simulink model "new5"  (R2025a)
settings: Solver=VariableStepAuto  StartTime=0.0  StopTime=20  RelTol=1e-3
undefined symbols (not defined in the file): g, Rs, Rsl, Rw, Ry
libraries: fl_lib x41, ee_lib x10, nesl_utility x10, slpidlib x3, spsFirstOrderFilterLib x2, spsabctodq0Lib x1
settings Model: SimulationMode=accelerator  Creator=maska  LastModifiedBy=maska

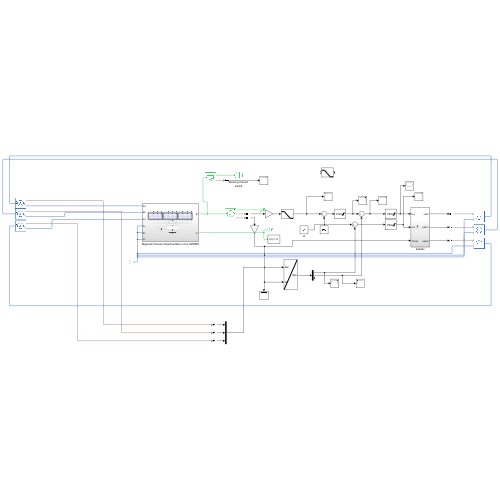
[thumbnail: Simulink's stored preview of the top-level diagram]
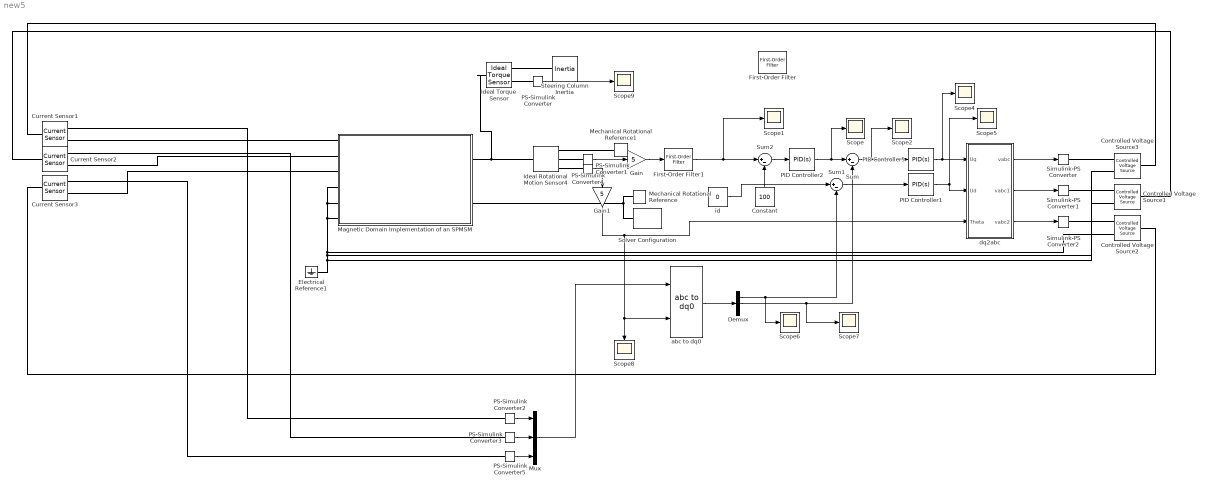
== system new5 ==
  Constant : Constant  Value=100
  Controlled Voltage Source1 : fl_lib/Electrical/Electrical Sources/Controlled Voltage Source
  Controlled Voltage Source2 : fl_lib/Electrical/Electrical Sources/Controlled Voltage Source
  Controlled Voltage Source3 : fl_lib/Electrical/Electrical Sources/Controlled Voltage Source
  Current Sensor1 : fl_lib/Electrical/Electrical Sensors/Current Sensor
  Current Sensor2 : fl_lib/Electrical/Electrical Sensors/Current Sensor
  Current Sensor3 : fl_lib/Electrical/Electrical Sensors/Current Sensor
  Demux : Demux  Outputs=3
  Electrical Reference1 : fl_lib/Electrical/Electrical Elements/Electrical Reference
  First-Order Filter : spsFirstOrderFilterLib/First-Order Filter  FilterType=Lowpass  Tc=0.05  Ts=0  Initialize=on  Vac_Init=[0, 0, 60]  Vdc_Init=0  PlotResponse=off  FreqRange="[0,  200,  1]"
  First-Order Filter1 : spsFirstOrderFilterLib/First-Order Filter  FilterType=Lowpass  Tc=0.1  Ts=0  Initialize=on  Vac_Init=[0, 0, 60]  Vdc_Init=0  PlotResponse=off  FreqRange="[0,  200,  1]"
  Gain : Gain  Gain=5
  Gain1 : Gain  Gain=5
  Ideal Rotational Motion Sensor4 : fl_lib/Mechanical/Mechanical Sensors/Ideal Rotational Motion Sensor  reference=foundation.enum.MeasurementReference.difference  acceleration_port=false  velocity_port=true  position_port=true  wrap_angle=false  offset=0 rad
  Ideal Torque Sensor : fl_lib/Mechanical/Mechanical Sensors/Ideal Torque Sensor
  Magnetic Domain Implementation of an SPMSM : Subsystem
  Mechanical Rotational Reference : fl_lib/Mechanical/Rotational Elements/Mechanical Rotational Reference
  Mechanical Rotational Reference1 : fl_lib/Mechanical/Rotational Elements/Mechanical Rotational Reference
  Mux : Mux  Inputs=3
  PID Controller1 : slpidlib/PID Controller  Controller=PID  Form=Parallel  TimeDomain=Continuous-time  UseExternalTs=off  SampleTime=-1  IntegratorMethod=Forward Euler  FilterMethod=Forward Euler  ControllerParametersSource=internal  P=1.3  I=0.3  UseKiTs=off  D=0  UseExternalDerivativeSource=off  N=100  UseFilter=on  TunerSelectOption=Transfer Function Based (PID Tuner App)  InitialConditionSource=internal  InitialConditionForIntegrator=0  InitialConditionForFilter=0  DifferentiatorICPrevScaledInput=0  ExternalReset=none  TrackingMode=off  Kt=1  LimitOutput=on  SatLimitsSource=internal  UpperSaturationLimit=1000  LowerSaturationLimit=-1000  LinearizeAsGain=on  AntiWindupMode=none  Kb=1  LimitIntegrator=off  UpperIntegratorSaturationLimit=inf  LowerIntegratorSaturationLimit=-inf  POutMin=[]  POutMax=[]  IOutMin=[]  IOutMax=[]  DOutMin=[]  DOutMax=[]  NOutMin=[]  NOutMax=[]  SumOutMin=[]  SumOutMax=[]  SaturationOutMin=[]  SaturationOutMax=[]  PParamMin=[]  PParamMax=[]  IParamMin=[]  IParamMax=[]  DParamMin=[]  DParamMax=[]  NParamMin=[]  NParamMax=[]  KbParamMin=[]  KbParamMax=[]  KtParamMin=[]  KtParamMax=[]  KbOutMin=[]  KbOutMax=[]  KtOutMin=[]  KtOutMax=[]  IntegratorOutMin=[]  IntegratorOutMax=[]  FilterOutMin=[]  FilterOutMax=[]  SumI1OutMin=[]  SumI1OutMax=[]  SumI2OutMin=[]  SumI2OutMax=[]  SumI3OutMin=[]  SumI3OutMax=[]  SumI4OutMin=[]  SumI4OutMax=[]  SumDOutMin=[]  SumDOutMax=[]  DifferentiatorOutMin=[]  DifferentiatorOutMax=[]  FilterDiffOutCoefMin=[]  FilterDiffOutCoefMax=[]  ReciprocalOutMin=[]  ReciprocalOutMax=[]  SumDenOutMin=[]  SumDenOutMax=[]  SumNumOutMin=[]  SumNumOutMax=[]  DivideOutMin=[]  DivideOutMax=[]  UdiffTsProdOutMin=[]  UdiffTsProdOutMax=[]  NTsProdOutMin=[]  NTsProdOutMax=[]  UintegralTsProdOutMin=[]  UintegralTsProdOutMax=[]  UngainTsProdOutMin=[]  UngainTsProdOutMax=[]  ClampingZeroOutDataTypeStr=Inherit: Inherit via back propagation  ClampingZeroOutMin=[]  ClampingZeroOutMax=[]  FilterDenConstantOutDataTypeStr=Inherit: Inherit via back propagation  FilterDenConstantOutMin=[]  FilterDenConstantOutMax=[]  PCopyOutDataTypeStr=Inherit: Inherit via back propagation  PCopyOutMin=[]  PCopyOutMax=[]  NCopyOutDataTypeStr=Inherit: Inherit via back propagation  NCopyOutMin=[]  NCopyOutMax=[]  IntegratorContinuousStateAttributes=''  IntegratorStateMustResolveToSignalObject=off  IntegratorRTWStateStorageClass=Auto  FilterContinuousStateAttributes=''  FilterStateMustResolveToSignalObject=off  FilterRTWStateStorageClass=Auto  ParallelPVariant=InternalParameters  IdealPVariant=Disabled  IVariant=InternalParameters  DVariant=InternalParameters  IntegratorVariant=Continuous  SatVariant=Enabled  AWVariant=Passthrough  PCopyVariant=Disabled  TRVariant=Disabled  FdbkBlocksVariant=Forward  IdealPFdbkVariant=Disabled  SatFdbkVariant=Disabled  DerivativeFilterVariant=ContFilter  NVariant=InternalParameters  NCopyVariant=Disabled  FilterICVariant=InternalICsFilter  IntegratorICVariant=InternalICs  ExternalResetVariant=Disabled  TRSumVariant=Passthrough  SumFdbkVariant=Disabled  SumVariant=Sum_PID  TsampFilterVariant=InternalTs  TsampNgainVariant=Passthrough  TsampIntegralVariant=Disabled_SignalSpec  ExternalSaturationOutDataTypeStr=Inherit: Same as second input  DerivativeSourceVariant=ErrorSignal  PreIntVariant=InternalPreInt
  PID Controller2 : slpidlib/PID Controller  Controller=PID  Form=Parallel  TimeDomain=Continuous-time  UseExternalTs=off  SampleTime=-1  IntegratorMethod=Forward Euler  FilterMethod=Forward Euler  ControllerParametersSource=internal  P=0.02  I=0.007  UseKiTs=off  D=0  UseExternalDerivativeSource=off  N=100  UseFilter=on  TunerSelectOption=Transfer Function Based (PID Tuner App)  InitialConditionSource=internal  InitialConditionForIntegrator=0  InitialConditionForFilter=0  DifferentiatorICPrevScaledInput=0  ExternalReset=none  TrackingMode=off  Kt=1  LimitOutput=on  SatLimitsSource=internal  UpperSaturationLimit=100  LowerSaturationLimit=-100  LinearizeAsGain=on  AntiWindupMode=none  Kb=1  LimitIntegrator=off  UpperIntegratorSaturationLimit=inf  LowerIntegratorSaturationLimit=-inf  POutMin=[]  POutMax=[]  IOutMin=[]  IOutMax=[]  DOutMin=[]  DOutMax=[]  NOutMin=[]  NOutMax=[]  SumOutMin=[]  SumOutMax=[]  SaturationOutMin=[]  SaturationOutMax=[]  PParamMin=[]  PParamMax=[]  IParamMin=[]  IParamMax=[]  DParamMin=[]  DParamMax=[]  NParamMin=[]  NParamMax=[]  KbParamMin=[]  KbParamMax=[]  KtParamMin=[]  KtParamMax=[]  KbOutMin=[]  KbOutMax=[]  KtOutMin=[]  KtOutMax=[]  IntegratorOutMin=[]  IntegratorOutMax=[]  FilterOutMin=[]  FilterOutMax=[]  SumI1OutMin=[]  SumI1OutMax=[]  SumI2OutMin=[]  SumI2OutMax=[]  SumI3OutMin=[]  SumI3OutMax=[]  SumI4OutMin=[]  SumI4OutMax=[]  SumDOutMin=[]  SumDOutMax=[]  DifferentiatorOutMin=[]  DifferentiatorOutMax=[]  FilterDiffOutCoefMin=[]  FilterDiffOutCoefMax=[]  ReciprocalOutMin=[]  ReciprocalOutMax=[]  SumDenOutMin=[]  SumDenOutMax=[]  SumNumOutMin=[]  SumNumOutMax=[]  DivideOutMin=[]  DivideOutMax=[]  UdiffTsProdOutMin=[]  UdiffTsProdOutMax=[]  NTsProdOutMin=[]  NTsProdOutMax=[]  UintegralTsProdOutMin=[]  UintegralTsProdOutMax=[]  UngainTsProdOutMin=[]  UngainTsProdOutMax=[]  ClampingZeroOutDataTypeStr=Inherit: Inherit via back propagation  ClampingZeroOutMin=[]  ClampingZeroOutMax=[]  FilterDenConstantOutDataTypeStr=Inherit: Inherit via back propagation  FilterDenConstantOutMin=[]  FilterDenConstantOutMax=[]  PCopyOutDataTypeStr=Inherit: Inherit via back propagation  PCopyOutMin=[]  PCopyOutMax=[]  NCopyOutDataTypeStr=Inherit: Inherit via back propagation  NCopyOutMin=[]  NCopyOutMax=[]  IntegratorContinuousStateAttributes=''  IntegratorStateMustResolveToSignalObject=off  IntegratorRTWStateStorageClass=Auto  FilterContinuousStateAttributes=''  FilterStateMustResolveToSignalObject=off  FilterRTWStateStorageClass=Auto  ParallelPVariant=InternalParameters  IdealPVariant=Disabled  IVariant=InternalParameters  DVariant=InternalParameters  IntegratorVariant=Continuous  SatVariant=Enabled  AWVariant=Passthrough  PCopyVariant=Disabled  TRVariant=Disabled  FdbkBlocksVariant=Forward  IdealPFdbkVariant=Disabled  SatFdbkVariant=Disabled  DerivativeFilterVariant=ContFilter  NVariant=InternalParameters  NCopyVariant=Disabled  FilterICVariant=InternalICsFilter  IntegratorICVariant=InternalICs  ExternalResetVariant=Disabled  TRSumVariant=Passthrough  SumFdbkVariant=Disabled  SumVariant=Sum_PID  TsampFilterVariant=InternalTs  TsampNgainVariant=Passthrough  TsampIntegralVariant=Disabled_SignalSpec  ExternalSaturationOutDataTypeStr=Inherit: Same as second input  DerivativeSourceVariant=ErrorSignal  PreIntVariant=InternalPreInt
  PID Controller5 : slpidlib/PID Controller  Controller=PID  Form=Parallel  TimeDomain=Continuous-time  UseExternalTs=off  SampleTime=-1  IntegratorMethod=Forward Euler  FilterMethod=Forward Euler  ControllerParametersSource=internal  P=1.3  I=0.3  UseKiTs=off  D=0  UseExternalDerivativeSource=off  N=100  UseFilter=on  TunerSelectOption=Transfer Function Based (PID Tuner App)  InitialConditionSource=internal  InitialConditionForIntegrator=0  InitialConditionForFilter=0  DifferentiatorICPrevScaledInput=0  ExternalReset=none  TrackingMode=off  Kt=1  LimitOutput=on  SatLimitsSource=internal  UpperSaturationLimit=1000  LowerSaturationLimit=-1000  LinearizeAsGain=on  AntiWindupMode=none  Kb=1  LimitIntegrator=off  UpperIntegratorSaturationLimit=inf  LowerIntegratorSaturationLimit=-inf  POutMin=[]  POutMax=[]  IOutMin=[]  IOutMax=[]  DOutMin=[]  DOutMax=[]  NOutMin=[]  NOutMax=[]  SumOutMin=[]  SumOutMax=[]  SaturationOutMin=[]  SaturationOutMax=[]  PParamMin=[]  PParamMax=[]  IParamMin=[]  IParamMax=[]  DParamMin=[]  DParamMax=[]  NParamMin=[]  NParamMax=[]  KbParamMin=[]  KbParamMax=[]  KtParamMin=[]  KtParamMax=[]  KbOutMin=[]  KbOutMax=[]  KtOutMin=[]  KtOutMax=[]  IntegratorOutMin=[]  IntegratorOutMax=[]  FilterOutMin=[]  FilterOutMax=[]  SumI1OutMin=[]  SumI1OutMax=[]  SumI2OutMin=[]  SumI2OutMax=[]  SumI3OutMin=[]  SumI3OutMax=[]  SumI4OutMin=[]  SumI4OutMax=[]  SumDOutMin=[]  SumDOutMax=[]  DifferentiatorOutMin=[]  DifferentiatorOutMax=[]  FilterDiffOutCoefMin=[]  FilterDiffOutCoefMax=[]  ReciprocalOutMin=[]  ReciprocalOutMax=[]  SumDenOutMin=[]  SumDenOutMax=[]  SumNumOutMin=[]  SumNumOutMax=[]  DivideOutMin=[]  DivideOutMax=[]  UdiffTsProdOutMin=[]  UdiffTsProdOutMax=[]  NTsProdOutMin=[]  NTsProdOutMax=[]  UintegralTsProdOutMin=[]  UintegralTsProdOutMax=[]  UngainTsProdOutMin=[]  UngainTsProdOutMax=[]  ClampingZeroOutDataTypeStr=Inherit: Inherit via back propagation  ClampingZeroOutMin=[]  ClampingZeroOutMax=[]  FilterDenConstantOutDataTypeStr=Inherit: Inherit via back propagation  FilterDenConstantOutMin=[]  FilterDenConstantOutMax=[]  PCopyOutDataTypeStr=Inherit: Inherit via back propagation  PCopyOutMin=[]  PCopyOutMax=[]  NCopyOutDataTypeStr=Inherit: Inherit via back propagation  NCopyOutMin=[]  NCopyOutMax=[]  IntegratorContinuousStateAttributes=''  IntegratorStateMustResolveToSignalObject=off  IntegratorRTWStateStorageClass=Auto  FilterContinuousStateAttributes=''  FilterStateMustResolveToSignalObject=off  FilterRTWStateStorageClass=Auto  ParallelPVariant=InternalParameters  IdealPVariant=Disabled  IVariant=InternalParameters  DVariant=InternalParameters  IntegratorVariant=Continuous  SatVariant=Enabled  AWVariant=Passthrough  PCopyVariant=Disabled  TRVariant=Disabled  FdbkBlocksVariant=Forward  IdealPFdbkVariant=Disabled  SatFdbkVariant=Disabled  DerivativeFilterVariant=ContFilter  NVariant=InternalParameters  NCopyVariant=Disabled  FilterICVariant=InternalICsFilter  IntegratorICVariant=InternalICs  ExternalResetVariant=Disabled  TRSumVariant=Passthrough  SumFdbkVariant=Disabled  SumVariant=Sum_PID  TsampFilterVariant=InternalTs  TsampNgainVariant=Passthrough  TsampIntegralVariant=Disabled_SignalSpec  ExternalSaturationOutDataTypeStr=Inherit: Same as second input  DerivativeSourceVariant=ErrorSignal  PreIntVariant=InternalPreInt
  PS-Simulink Converter{,1..5} (6 alike) : nesl_utility/PS-Simulink Converter  PhysicalDomain=network_engine_domain  SubClassName=ps_output  LeftPortType=input  RightPortType=output  PseudoPeriodic=off  Frequencies=[]  VectorFormat=inherit  Unit=inherit  AffineConversion=off
  Scope{,1..2,4..9} (9 alike) : Scope
      Scope settings: ActiveDisplayYMinimum=-5.8023563752218168  ActiveDisplayYMaximum=2.2185184248670029
      Scope1 settings: ActiveDisplayYMinimum=-13.403661054802928  ActiveDisplayYMaximum=120.63294949322639
      Scope2 settings: ActiveDisplayYMinimum=-86.659334603066554  ActiveDisplayYMaximum=127.58889127165779  DataLoggingVariableName=ScopeData2
      Scope4 settings: ActiveDisplayYMinimum=-20.812297134459023  ActiveDisplayYMaximum=19.890291636244882  DataLoggingVariableName=ScopeData4
      Scope5 settings: ActiveDisplayYMinimum=24.495382360291835  ActiveDisplayYMaximum=76.354132200573616  DataLoggingVariableName=ScopeData5
      Scope6 settings: ActiveDisplayYMinimum=-3358.5009916772633  ActiveDisplayYMaximum=3314.8973874888006  DataLoggingVariableName=ScopeData6
      Scope7 settings: ActiveDisplayYMinimum=-2.8426588150958878  ActiveDisplayYMaximum=1.0409285736394622  DataLoggingVariableName=ScopeData7
      Scope8 settings: ActiveDisplayYMinimum=10.636225564991161  ActiveDisplayYMaximum=10.664194284729955  DataLoggingVariableName=ScopeData8
      Scope9 settings: ActiveDisplayYMinimum=-2.6472347032555867  ActiveDisplayYMaximum=2.6879452789265237  DataLoggingVariableName=ScopeData9
  Simulink-PS Converter : nesl_utility/Simulink-PS Converter  PhysicalDomain=network_engine_domain  SubClassName=ps_input  LeftPortType=input  RightPortType=output  PseudoPeriodic=off  Frequencies=[]  NoiseDistribution=none  NoiseParameters=[]  Unit=1  AffineConversion=off  FilteringAndDerivatives=provide  SimscapeFilterOrder=1  InputFilterTimeConstant=0.001  UdotUserProvided=0
  Simulink-PS Converter1 : nesl_utility/Simulink-PS Converter  PhysicalDomain=network_engine_domain  SubClassName=ps_input  LeftPortType=input  RightPortType=output  PseudoPeriodic=off  Frequencies=[]  NoiseDistribution=none  NoiseParameters=[]  Unit=1  AffineConversion=off  FilteringAndDerivatives=provide  SimscapeFilterOrder=1  InputFilterTimeConstant=0.001  UdotUserProvided=0
  Simulink-PS Converter2 : nesl_utility/Simulink-PS Converter  PhysicalDomain=network_engine_domain  SubClassName=ps_input  LeftPortType=input  RightPortType=output  PseudoPeriodic=off  Frequencies=[]  NoiseDistribution=none  NoiseParameters=[]  Unit=1  AffineConversion=off  FilteringAndDerivatives=provide  SimscapeFilterOrder=1  InputFilterTimeConstant=0.001  UdotUserProvided=0
  Solver Configuration : nesl_utility/Solver Configuration  PhysicalDomain=network_engine_domain  SubClassName=solver  LeftPortType=input  RightPortType=generic  Tones=[]  Harmonics=[]  SimulateNoise=off  Profile=off  UseLocalSampling=off  EnableSwitchedLinearOptims=on  FrequencyDomain=off  UseCCode=off  RelTol=0.001  AbsTol=1e-06  MinStep=1e-09  ToWorkspace=off  RevertToSquareIcSolve=off  NumHomotopyIterations=100  PhasorMode=off  PhasorModeNumHarmonics=1  ConsistencySolver=NEWTON_FTOL  IndexReductionMethod=DerivativeReplacement  DoDC=off  ResidualTolerance=1e-09  ConsistencyTolSource=GLOBAL  ConsistencyAbsTol=0.001  ConsistencyRelTol=0.001  ConsistencyTolFactor=0.001  UseLocalSolver=off  LocalSolverChoice=NE_BACKWARD_EULER_ADVANCER  ResolveIndetEquations=on  FunctionEvalNumThread=1  LocalSolverSampleTime=0.0001  DoFixedCost=off  MaxNonlinIter=3  MaxModeIter=2  ComputeImpulses=off  ImpulseIterations=1  LinearAlgebra=auto  LinearAlgebraNumThread=0  EquationFormulation=NE_TIME_EF  DelaysMemoryBudget=1024  AutomaticFiltering=on  FilteringTimeConstant=0.001  PartitionStorageMethod=AS_NEEDED  PartitionMemoryBudget=1024  PartitionMethod=ROBUST  MultibodyUseLocalSolver=off  MultibodyLocalSolverChoice=ODE1  MultibodyLocalSolverSampleTime=0.001
  Steering Column Inertia : fl_lib/Mechanical/Rotational Elements/Inertia  inertia=1e-3 kg*m^2  num_ports=foundation.enum.numPorts2.one  w_specify=off  w_priority=High  w=0 rad/s  w_nominal_specify=off  w_nominal_value=1  w_nominal_unit=rad/s  t_specify=off  t_priority=High  t=0 N*m  t_nominal_specify=off  t_nominal_value=1  t_nominal_unit=N*m
      settings: LogSimulationData=on
  Sum : Sum  Inputs=|+-
  Sum1 : Sum  Inputs=|+-
  Sum2 : Sum  Inputs=|+-
  abc to dq0 : spsabctodq0Lib/abc to dq0  Alignment=90 degrees behind phase A axis
  dq2abc : Subsystem
  id : Constant  Value=0
  wires:
  PS-Simulink Converter2/1 -> Mux/1
  PID Controller2/1 -> Scope/1, Sum/1
  PID Controller1/1 -> dq2abc/2(Ud), Scope5/1
  PS-Simulink Converter4/1 -> Gain/1
  Demux/2 -> Scope7/1, Sum/2
  Mux/1 -> abc to dq0/1
  abc to dq0/1 -> Demux/1
  id/1 -> Sum1/1
  Constant/1 -> Sum2/2
  Gain1/1 -> abc to dq0/2, Scope8/1, dq2abc/3(Theta)
  PS-Simulink Converter/1 -> Scope9/1
  PID Controller5/1 -> Scope4/1, dq2abc/1(Uq)
  PS-Simulink Converter3/1 -> Mux/2
  PS-Simulink Converter1/1 -> Gain1/1
  Sum1/1 -> PID Controller1/1
  Sum2/1 -> PID Controller2/1
  PS-Simulink Converter5/1 -> Mux/3
  dq2abc/1(vabc) -> Simulink-PS Converter/1
  Sum/1 -> PID Controller5/1, Scope2/1
  Demux/1 -> Sum1/2, Scope6/1
  dq2abc/2(vabc1) -> Simulink-PS Converter1/1
  dq2abc/3(vabc2) -> Simulink-PS Converter2/1
  First-Order Filter1/1 -> Scope1/1, Sum2/1
  Gain/1 -> First-Order Filter1/1
  connections:
  Magnetic Domain Implementation of an SPMSM/RConn1 -- Ideal Rotational Motion Sensor4/LConn1 -- Ideal Torque Sensor/LConn1
  Magnetic Domain Implementation of an SPMSM/RConn2 -- Solver Configuration/RConn1 -- Mechanical Rotational Reference/LConn1
  Magnetic Domain Implementation of an SPMSM/LConn5 -- Magnetic Domain Implementation of an SPMSM/LConn4 -- Controlled Voltage Source3/RConn2 -- Electrical Reference1/LConn1 -- Controlled Voltage Source1/RConn2 -- Controlled Voltage Source2/RConn2 -- Magnetic Domain Implementation of an SPMSM/LConn6
  PS-Simulink Converter/LConn1 -- Ideal Torque Sensor/RConn2
  PS-Simulink Converter1/LConn1 -- Ideal Rotational Motion Sensor4/RConn3
  PS-Simulink Converter2/LConn1 -- Current Sensor1/RConn1
  PS-Simulink Converter3/LConn1 -- Current Sensor2/RConn1
  Ideal Rotational Motion Sensor4/RConn1 -- Mechanical Rotational Reference1/LConn1
  Steering Column Inertia/LConn1 -- Ideal Torque Sensor/RConn1
  Ideal Rotational Motion Sensor4/RConn2 -- PS-Simulink Converter4/LConn1
  PS-Simulink Converter5/LConn1 -- Current Sensor3/RConn1
  Controlled Voltage Source3/RConn1 -- Simulink-PS Converter/RConn1
  Simulink-PS Converter1/RConn1 -- Controlled Voltage Source1/RConn1
  Controlled Voltage Source2/RConn1 -- Simulink-PS Converter2/RConn1
  Current Sensor1/LConn1 -- Controlled Voltage Source3/LConn1
  Controlled Voltage Source1/LConn1 -- Current Sensor2/LConn1
  Controlled Voltage Source2/LConn1 -- Current Sensor3/LConn1
  Current Sensor1/RConn2 -- Magnetic Domain Implementation of an SPMSM/LConn1
  Current Sensor3/RConn2 -- Magnetic Domain Implementation of an SPMSM/LConn3
  Current Sensor2/RConn2 -- Magnetic Domain Implementation of an SPMSM/LConn2

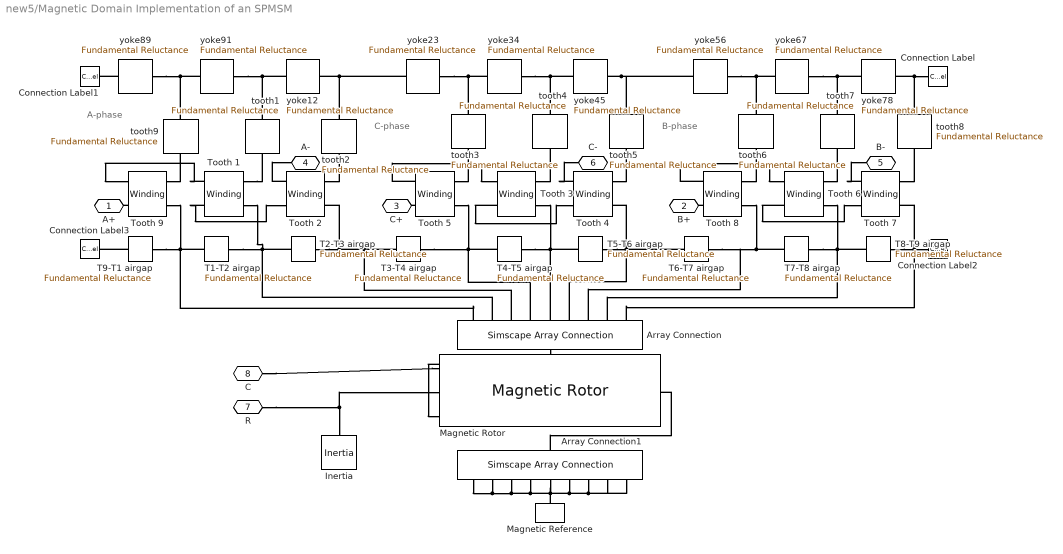
== system new5/Magnetic Domain Implementation of an SPMSM ==
  note: A-phase
  note: C-phase
  note: B-phase
  Array Connection : SimscapeArrayConnection  Domain=foundation.magnetic.magnetic  NumScalarElements=9
  Array Connection1 : SimscapeArrayConnection  Domain=foundation.magnetic.magnetic  NumScalarElements=9
  Connection Label : ConnectionLabel  Label=Y
  Connection Label1 : ConnectionLabel  Label=Y
  Connection Label2 : ConnectionLabel  Label=SL
  Connection Label3 : ConnectionLabel  Label=SL
  Inertia : fl_lib/Mechanical/Rotational Elements/Inertia  inertia=J kg*m^2  num_ports=foundation.enum.numPorts2.one  w_specify=on  w_priority=None  w=0 rad/s  w_nominal_specify=off  w_nominal_value=1  w_nominal_unit=rad/s  t_specify=off  t_priority=High  t=0 N*m  t_nominal_specify=off  t_nominal_value=1  t_nominal_unit=N*m
  Magnetic Reference : fl_lib/Magnetic/Magnetic Elements/Magnetic Reference
      settings: InternalSimscapePortConfiguration="{\"Bottom\":[],\"Left\":[{\"id\":\"M\",\"label\":\"\",\"type\":\"foundation.magnetic.magnetic\"}],\"Right\":[],\"Top\":[]}"
  Magnetic Rotor : ee_lib/Electromechanical/Magnetic Rotor  Nr=5  Ns=Ns  B0=B0 T  lm=lm mm  mur=1.05  g=g mm  r=r mm  l=l mm
      settings: InternalSimscapePortConfiguration="{\"Bottom\":[{\"id\":\"S\",\"label\":\"S\",\"type\":\"foundation.magnetic.magnetic\"}],\"Left\":[{\"id\":\"C\",\"label\":\"C\",\"type\":\"foundation.mechanical.rotational.rotational\"},{\"id\":\"R\",\"label\":\"R\",\"type\":\"foundation.mechanical.rotational.rotational\"}],\"Right\":[],\"Top\":[{\"id\":\"N\",\"label\":\"N\",\"type\":\"foundation.magnetic.magnetic\"}]}"
  T1-T2 airgap : fl_lib/Magnetic/Magnetic Elements/Fundamental Reluctance  R=Rsl 1/H  phi_specify=off  phi_priority=None  phi=0 Wb  phi_nominal_specify=off  phi_nominal_value=1  phi_nominal_unit=Wb  mmf_specify=off  mmf_priority=None  mmf=0 A  mmf_nominal_specify=off  mmf_nominal_value=1  mmf_nominal_unit=A
      settings: InternalSimscapePortConfiguration="{\"Bottom\":[],\"Left\":[{\"id\":\"N\",\"label\":\"N\",\"type\":\"foundation.magnetic.magnetic\"}],\"Right\":[{\"id\":\"S\",\"label\":\"S\",\"type\":\"foundation.magnetic.magnetic\"}],\"Top\":[]}"
  T2-T3 airgap : fl_lib/Magnetic/Magnetic Elements/Fundamental Reluctance  R=Rsl 1/H  phi_specify=off  phi_priority=None  phi=0 Wb  phi_nominal_specify=off  phi_nominal_value=1  phi_nominal_unit=Wb  mmf_specify=off  mmf_priority=None  mmf=0 A  mmf_nominal_specify=off  mmf_nominal_value=1  mmf_nominal_unit=A
      settings: InternalSimscapePortConfiguration="{\"Bottom\":[],\"Left\":[{\"id\":\"N\",\"label\":\"N\",\"type\":\"foundation.magnetic.magnetic\"}],\"Right\":[{\"id\":\"S\",\"label\":\"S\",\"type\":\"foundation.magnetic.magnetic\"}],\"Top\":[]}"
  T3-T4 airgap : fl_lib/Magnetic/Magnetic Elements/Fundamental Reluctance  R=Rsl 1/H  phi_specify=off  phi_priority=None  phi=0 Wb  phi_nominal_specify=off  phi_nominal_value=1  phi_nominal_unit=Wb  mmf_specify=off  mmf_priority=None  mmf=0 A  mmf_nominal_specify=off  mmf_nominal_value=1  mmf_nominal_unit=A
      settings: InternalSimscapePortConfiguration="{\"Bottom\":[],\"Left\":[{\"id\":\"N\",\"label\":\"N\",\"type\":\"foundation.magnetic.magnetic\"}],\"Right\":[{\"id\":\"S\",\"label\":\"S\",\"type\":\"foundation.magnetic.magnetic\"}],\"Top\":[]}"
  T4-T5 airgap : fl_lib/Magnetic/Magnetic Elements/Fundamental Reluctance  R=Rsl 1/H  phi_specify=off  phi_priority=None  phi=0 Wb  phi_nominal_specify=off  phi_nominal_value=1  phi_nominal_unit=Wb  mmf_specify=off  mmf_priority=None  mmf=0 A  mmf_nominal_specify=off  mmf_nominal_value=1  mmf_nominal_unit=A
      settings: InternalSimscapePortConfiguration="{\"Bottom\":[],\"Left\":[{\"id\":\"N\",\"label\":\"N\",\"type\":\"foundation.magnetic.magnetic\"}],\"Right\":[{\"id\":\"S\",\"label\":\"S\",\"type\":\"foundation.magnetic.magnetic\"}],\"Top\":[]}"
  T5-T6 airgap : fl_lib/Magnetic/Magnetic Elements/Fundamental Reluctance  R=Rsl 1/H  phi_specify=off  phi_priority=None  phi=0 Wb  phi_nominal_specify=off  phi_nominal_value=1  phi_nominal_unit=Wb  mmf_specify=off  mmf_priority=None  mmf=0 A  mmf_nominal_specify=off  mmf_nominal_value=1  mmf_nominal_unit=A
      settings: InternalSimscapePortConfiguration="{\"Bottom\":[],\"Left\":[{\"id\":\"N\",\"label\":\"N\",\"type\":\"foundation.magnetic.magnetic\"}],\"Right\":[{\"id\":\"S\",\"label\":\"S\",\"type\":\"foundation.magnetic.magnetic\"}],\"Top\":[]}"
  T6-T7 airgap : fl_lib/Magnetic/Magnetic Elements/Fundamental Reluctance  R=Rsl 1/H  phi_specify=off  phi_priority=None  phi=0 Wb  phi_nominal_specify=off  phi_nominal_value=1  phi_nominal_unit=Wb  mmf_specify=off  mmf_priority=None  mmf=0 A  mmf_nominal_specify=off  mmf_nominal_value=1  mmf_nominal_unit=A
      settings: InternalSimscapePortConfiguration="{\"Bottom\":[],\"Left\":[{\"id\":\"N\",\"label\":\"N\",\"type\":\"foundation.magnetic.magnetic\"}],\"Right\":[{\"id\":\"S\",\"label\":\"S\",\"type\":\"foundation.magnetic.magnetic\"}],\"Top\":[]}"
  T7-T8 airgap : fl_lib/Magnetic/Magnetic Elements/Fundamental Reluctance  R=Rsl 1/H  phi_specify=off  phi_priority=None  phi=0 Wb  phi_nominal_specify=off  phi_nominal_value=1  phi_nominal_unit=Wb  mmf_specify=off  mmf_priority=None  mmf=0 A  mmf_nominal_specify=off  mmf_nominal_value=1  mmf_nominal_unit=A
      settings: InternalSimscapePortConfiguration="{\"Bottom\":[],\"Left\":[{\"id\":\"N\",\"label\":\"N\",\"type\":\"foundation.magnetic.magnetic\"}],\"Right\":[{\"id\":\"S\",\"label\":\"S\",\"type\":\"foundation.magnetic.magnetic\"}],\"Top\":[]}"
  T8-T9 airgap : fl_lib/Magnetic/Magnetic Elements/Fundamental Reluctance  R=Rsl 1/H  phi_specify=off  phi_priority=None  phi=0 Wb  phi_nominal_specify=off  phi_nominal_value=1  phi_nominal_unit=Wb  mmf_specify=off  mmf_priority=None  mmf=0 A  mmf_nominal_specify=off  mmf_nominal_value=1  mmf_nominal_unit=A
      settings: InternalSimscapePortConfiguration="{\"Bottom\":[],\"Left\":[{\"id\":\"N\",\"label\":\"N\",\"type\":\"foundation.magnetic.magnetic\"}],\"Right\":[{\"id\":\"S\",\"label\":\"S\",\"type\":\"foundation.magnetic.magnetic\"}],\"Top\":[]}"
  T9-T1 airgap : fl_lib/Magnetic/Magnetic Elements/Fundamental Reluctance  R=Rsl 1/H  phi_specify=off  phi_priority=None  phi=0 Wb  phi_nominal_specify=off  phi_nominal_value=1  phi_nominal_unit=Wb  mmf_specify=off  mmf_priority=None  mmf=0 A  mmf_nominal_specify=off  mmf_nominal_value=1  mmf_nominal_unit=A
      settings: InternalSimscapePortConfiguration="{\"Bottom\":[],\"Left\":[{\"id\":\"N\",\"label\":\"N\",\"type\":\"foundation.magnetic.magnetic\"}],\"Right\":[{\"id\":\"S\",\"label\":\"S\",\"type\":\"foundation.magnetic.magnetic\"}],\"Top\":[]}"
  Tooth {1..9} (9 alike) : ee_lib/Passive/Winding  Nw=Nws  Rw=Rw/3 Ohm  Rl=inf 1/H  Gw=gWinding 1/Ohm  thermalPort=simscape.enum.thermaleffects.omit  alpha=3.93e-3 1/K  Tmeas=25 degC  winding_thermal_mass=100 J/K  T_specify=off  T_priority=None  T=25 degC  T_nominal_specify=off  T_nominal_value=1  T_nominal_unit=degC  i_specify=off  i_priority=None  i=0 A  i_nominal_specify=off  i_nominal_value=1  i_nominal_unit=A  v_specify=off  v_priority=None  v=0 V  v_nominal_specify=off  v_nominal_value=1  v_nominal_unit=V  phi_specify=off  phi_priority=None  phi=0 Wb  phi_nominal_specify=off  phi_nominal_value=1  phi_nominal_unit=Wb  iterm_p_specify=off  iterm_p_priority=None  iterm_p=0 A  iterm_p_nominal_specify=off  iterm_p_nominal_value=1  iterm_p_nominal_unit=A  iterm_n_specify=off  iterm_n_priority=None  iterm_n=0 A  iterm_n_nominal_specify=off  iterm_n_nominal_value=1  iterm_n_nominal_unit=A  power_dissipated_specify=off  power_dissipated_priority=None  power_dissipated=0 W  power_dissipated_nominal_specify=off  power_dissipated_nominal_value=1  power_dissipated_nominal_unit=W
      settings: InternalSimscapePortConfiguration="{\"Bottom\":[],\"Left\":[{\"id\":\"p\",\"label\":\"+\",\"type\":\"foundation.electrical.electrical\"},{\"id\":\"n\",\"label\":\"-\",\"type\":\"foundation.electrical.electrical\"}],\"Right\":[{\"id\":\"N\",\"label\":\"N\",\"type\":\"foundation.magnetic.magnetic\"},{\"id\":\"S\",\"label\":\"S\",\"type\":\"foundation.magnetic.magnetic\"}],\"Top\":[]}"
  tooth{1..9} (9 alike) : fl_lib/Magnetic/Magnetic Elements/Fundamental Reluctance  R=Rs 1/H  phi_specify=off  phi_priority=None  phi=0 Wb  phi_nominal_specify=off  phi_nominal_value=1  phi_nominal_unit=Wb  mmf_specify=off  mmf_priority=None  mmf=0 A  mmf_nominal_specify=off  mmf_nominal_value=1  mmf_nominal_unit=A
      settings: InternalSimscapePortConfiguration="{\"Bottom\":[],\"Left\":[{\"id\":\"N\",\"label\":\"N\",\"type\":\"foundation.magnetic.magnetic\"}],\"Right\":[{\"id\":\"S\",\"label\":\"S\",\"type\":\"foundation.magnetic.magnetic\"}],\"Top\":[]}"
  yoke{12,23,34,45,56,67,78,89,91} (9 alike) : fl_lib/Magnetic/Magnetic Elements/Fundamental Reluctance  R=Ry 1/H  phi_specify=off  phi_priority=None  phi=0 Wb  phi_nominal_specify=off  phi_nominal_value=1  phi_nominal_unit=Wb  mmf_specify=off  mmf_priority=None  mmf=0 A  mmf_nominal_specify=off  mmf_nominal_value=1  mmf_nominal_unit=A
      settings: InternalSimscapePortConfiguration="{\"Bottom\":[],\"Left\":[{\"id\":\"N\",\"label\":\"N\",\"type\":\"foundation.magnetic.magnetic\"}],\"Right\":[{\"id\":\"S\",\"label\":\"S\",\"type\":\"foundation.magnetic.magnetic\"}],\"Top\":[]}"
  A+ : PMIOPort  Side=Left
  B+ : PMIOPort  Port=2  Side=Left
  C+ : PMIOPort  Port=3  Side=Left
  A- : PMIOPort  Port=4  Side=Left
  B- : PMIOPort  Port=5  Side=Left
  C- : PMIOPort  Port=6  Side=Left
  R : PMIOPort  Port=7  Side=Right
  C : PMIOPort  Port=8  Side=Right
  connections:
  yoke91/RConn1 -- yoke12/LConn1 -- tooth1/LConn1
  Array Connection/LConn2 -- Tooth 1/RConn2 -- T2-T3 airgap/LConn1 -- T1-T2 airgap/RConn1
  T3-T4 airgap/LConn1 -- Array Connection/LConn3 -- Tooth 2/RConn2 -- T2-T3 airgap/RConn1
  Tooth 2/RConn1 -- tooth2/RConn1
  yoke91/LConn1 -- yoke89/RConn1 -- tooth9/LConn1
  yoke89/LConn1 -- Connection Label1/LConn1
  T9-T1 airgap/LConn1 -- Connection Label3/LConn1
  Tooth 9/LConn2 -- A+/RConn1
  Tooth 1/LConn1 -- Tooth 9/LConn1
  Tooth 1/LConn2 -- Tooth 2/LConn2
  Tooth 2/LConn1 -- A-/RConn1
  Tooth 9/RConn2 -- Array Connection/LConn1 -- T9-T1 airgap/RConn1 -- T1-T2 airgap/LConn1
  yoke45/LConn1 -- yoke34/RConn1 -- tooth4/LConn1
  Tooth 3/RConn2 -- Array Connection/LConn5 -- T5-T6 airgap/LConn1 -- T4-T5 airgap/RConn1
  T6-T7 airgap/LConn1 -- Array Connection/LConn6 -- T5-T6 airgap/RConn1 -- Tooth 4/RConn2
  yoke34/LConn1 -- yoke23/RConn1 -- tooth3/LConn1
  R/RConn1 -- Inertia/LConn1 -- Magnetic Rotor/LConn2
  Tooth 5/RConn2 -- Array Connection/LConn4 -- T3-T4 airgap/RConn1 -- T4-T5 airgap/LConn1
  yoke45/RConn1 -- yoke56/LConn1 -- tooth5/LConn1
  Tooth 5/LConn2 -- C+/RConn1
  Tooth 3/LConn2 -- Tooth 4/LConn2
  Tooth 5/LConn1 -- Tooth 3/LConn1
  Tooth 4/LConn1 -- C-/RConn1
  yoke78/LConn1 -- yoke67/RConn1 -- tooth7/LConn1
  Tooth 6/RConn2 -- Array Connection/LConn8 -- T8-T9 airgap/LConn1 -- T7-T8 airgap/RConn1
  T8-T9 airgap/RConn1 -- Array Connection/LConn9 -- Connection Label2/LConn1 -- Tooth 7/RConn2
  yoke67/LConn1 -- yoke56/RConn1 -- tooth6/LConn1
  Tooth 8/RConn2 -- Array Connection/LConn7 -- T6-T7 airgap/RConn1 -- T7-T8 airgap/LConn1
  C/RConn1 -- Magnetic Rotor/LConn1
  tooth8/LConn1 -- yoke78/RConn1 -- Connection Label/LConn1
  Tooth 8/LConn2 -- B+/RConn1
  Tooth 8/LConn1 -- Tooth 6/LConn1
  Tooth 6/LConn2 -- Tooth 7/LConn2
  Tooth 7/LConn1 -- B-/RConn1
  Tooth 1/RConn1 -- tooth1/RConn1
  yoke23/LConn1 -- tooth2/LConn1 -- yoke12/RConn1
  Tooth 5/RConn1 -- tooth3/RConn1
  Tooth 3/RConn1 -- tooth4/RConn1
  Tooth 4/RConn1 -- tooth5/RConn1
  Tooth 8/RConn1 -- tooth6/RConn1
  Tooth 6/RConn1 -- tooth7/RConn1
  Tooth 9/RConn1 -- tooth9/RConn1
  Tooth 7/RConn1 -- tooth8/RConn1
  Array Connection/RConn1 -- Magnetic Rotor/LConn3
  Array Connection1/RConn1 -- Magnetic Rotor/RConn1
  Array Connection1/LConn2 -- Array Connection1/LConn1 -- Array Connection1/LConn3 -- Array Connection1/LConn4 -- Magnetic Reference/LConn1 -- Array Connection1/LConn5 -- Array Connection1/LConn6 -- Array Connection1/LConn7 -- Array Connection1/LConn9 -- Array Connection1/LConn8

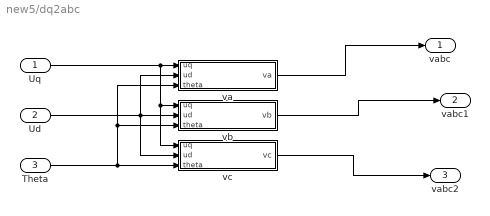
== system new5/dq2abc ==
  Uq : Inport
  Ud : Inport  Port=2
  Theta : Inport  Port=3
  va : Subsystem
  vb : Subsystem
  vc : Subsystem
  vabc : Outport  VectorParamsAs1DForOutWhenUnconnected=off
  vabc1 : Outport  Port=2  VectorParamsAs1DForOutWhenUnconnected=off
  vabc2 : Outport  Port=3  VectorParamsAs1DForOutWhenUnconnected=off
  wires:
  Ud/1 -> va/2(ud), vb/2(ud), vc/2(ud)
  Uq/1 -> vc/1(uq), vb/1(uq), va/1(uq)
  Theta/1 -> va/3(theta), vb/3(theta), vc/3(theta)
  va/1(va) -> vabc/1
  vb/1(vb) -> vabc1/1
  vc/1(vc) -> vabc2/1

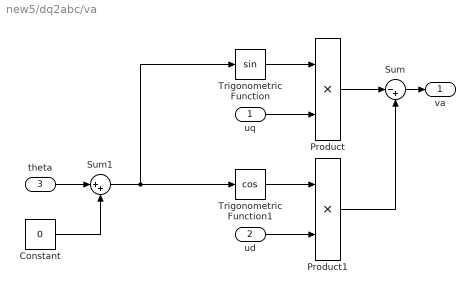
== system new5/dq2abc/va ==
  uq : Inport
  ud : Inport  Port=2
  theta : Inport  Port=3
  Constant : Constant  Value=0
  Product : Product
  Product1 : Product
  Sum : Sum  Inputs=|-+
  Sum1 : Sum  Inputs=|++
  Trigonometric Function : Trigonometry
  Trigonometric Function1 : Trigonometry  Operator=cos
  va : Outport  VectorParamsAs1DForOutWhenUnconnected=off
  wires:
  Product1/1 -> Sum/2
  Product/1 -> Sum/1
  ud/1 -> Product1/2
  Trigonometric Function/1 -> Product/1
  Trigonometric Function1/1 -> Product1/1
  Sum/1 -> va/1
  uq/1 -> Product/2
  Constant/1 -> Sum1/2
  theta/1 -> Sum1/1
  Sum1/1 -> Trigonometric Function1/1, Trigonometric Function/1

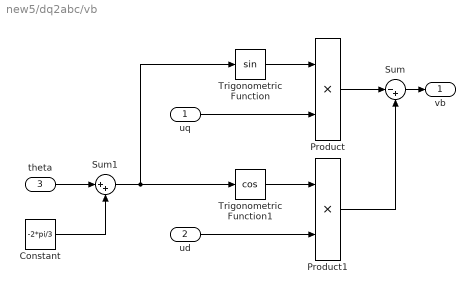
== system new5/dq2abc/vb ==
  uq : Inport
  ud : Inport  Port=2
  theta : Inport  Port=3
  Constant : Constant  Value=-2*pi/3
  Product : Product
  Product1 : Product
  Sum : Sum  Inputs=|-+
  Sum1 : Sum  Inputs=|++
  Trigonometric Function : Trigonometry
  Trigonometric Function1 : Trigonometry  Operator=cos
  vb : Outport  VectorParamsAs1DForOutWhenUnconnected=off
  wires:
  Product1/1 -> Sum/2
  Product/1 -> Sum/1
  ud/1 -> Product1/2
  Trigonometric Function/1 -> Product/1
  Trigonometric Function1/1 -> Product1/1
  Sum/1 -> vb/1
  uq/1 -> Product/2
  Constant/1 -> Sum1/2
  theta/1 -> Sum1/1
  Sum1/1 -> Trigonometric Function1/1, Trigonometric Function/1

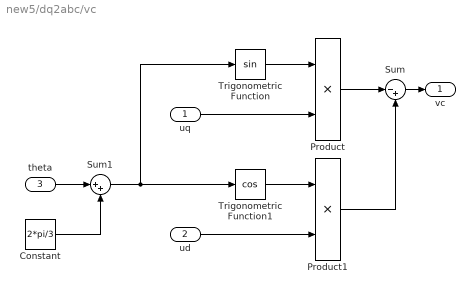
== system new5/dq2abc/vc ==
  uq : Inport
  ud : Inport  Port=2
  theta : Inport  Port=3
  Constant : Constant  Value=2*pi/3
  Product : Product
  Product1 : Product
  Sum : Sum  Inputs=|-+
  Sum1 : Sum  Inputs=|++
  Trigonometric Function : Trigonometry
  Trigonometric Function1 : Trigonometry  Operator=cos
  vc : Outport  VectorParamsAs1DForOutWhenUnconnected=off
  wires:
  Product1/1 -> Sum/2
  Product/1 -> Sum/1
  ud/1 -> Product1/2
  Trigonometric Function/1 -> Product/1
  Trigonometric Function1/1 -> Product1/1
  Sum/1 -> vc/1
  uq/1 -> Product/2
  Constant/1 -> Sum1/2
  theta/1 -> Sum1/1
  Sum1/1 -> Trigonometric Function1/1, Trigonometric Function/1
